simulink model "Zad1_Adasiak"  (R2020b)
settings: Solver=VariableStepAuto  StartTime=0.0  StopTime=0.0  RelTol=1e-3
undefined symbols (not defined in the file): H, W
libraries: CPOiS_SourcesSinks x10, CPOiS_LinearTransforms x4, CPOiS_DataManipulation_DataTypeConversion x4, CPOiS_General x1
settings Model: Creator=Krystian  LastModifiedBy=wadasiak

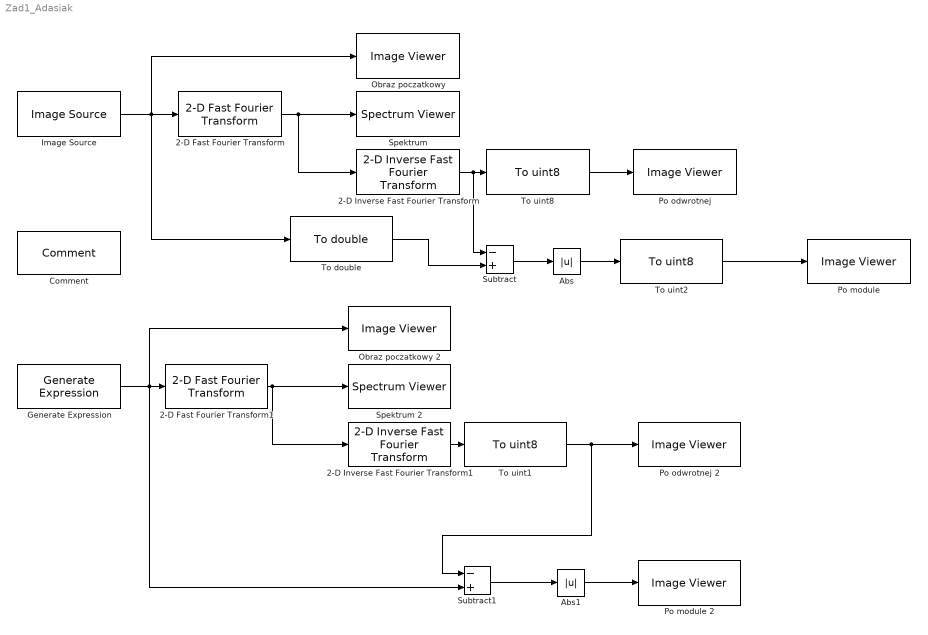
== system Zad1_Adasiak ==
  2-D Fast Fourier Transform : CPOiS_LinearTransforms/2-D Fast Fourier Transform
      settings: SourceProductName=CPOiS - Digital image and signal processing
  2-D Fast Fourier Transform1 : CPOiS_LinearTransforms/2-D Fast Fourier Transform
      settings: SourceProductName=CPOiS - Digital image and signal processing
  2-D Inverse Fast Fourier Transform : CPOiS_LinearTransforms/2-D Inverse Fast  Fourier Transform
      settings: SourceProductName=CPOiS - Digital image and signal processing
  2-D Inverse Fast Fourier Transform1 : CPOiS_LinearTransforms/2-D Inverse Fast  Fourier Transform
      settings: SourceProductName=CPOiS - Digital image and signal processing
  Abs : Abs
  Abs1 : Abs
  Comment : CPOiS_General/Comment
      settings: SourceProductName=CPOiS - Digital image and signal processing
  Generate Expression : CPOiS_SourcesSinks/Generate Expression  Width=256  Height=256  Expression=50.*(sin(W)+sin(2*H)+2)
      settings: SourceProductName=CPOiS - Digital image and signal processing
  Image Source : CPOiS_SourcesSinks/Image Source  FileSelection=marine.png
      settings: SourceProductName=CPOiS - Digital image and signal processing
  Obraz poczatkowy : CPOiS_SourcesSinks/Image Viewer
      settings: SourceProductName=CPOiS - Digital image and signal processing
  Obraz poczatkowy 2 : CPOiS_SourcesSinks/Image Viewer
      settings: SourceProductName=CPOiS - Digital image and signal processing
  Po module : CPOiS_SourcesSinks/Image Viewer
      settings: SourceProductName=CPOiS - Digital image and signal processing
  Po module 2 : CPOiS_SourcesSinks/Image Viewer
      settings: SourceProductName=CPOiS - Digital image and signal processing
  Po odwrotnej : CPOiS_SourcesSinks/Image Viewer
      settings: SourceProductName=CPOiS - Digital image and signal processing
  Po odwrotnej 2 : CPOiS_SourcesSinks/Image Viewer
      settings: SourceProductName=CPOiS - Digital image and signal processing
  Spektrum : CPOiS_SourcesSinks/Spectrum Viewer
      settings: SourceProductName=CPOiS - Digital image and signal processing
  Spektrum 2 : CPOiS_SourcesSinks/Spectrum Viewer
      settings: SourceProductName=CPOiS - Digital image and signal processing
  Subtract : Sum  Inputs=-+
  Subtract1 : Sum  Inputs=-+
  To double : CPOiS_DataManipulation_DataTypeConversion/To double
      settings: SourceProductName=CPOiS - Digital image and signal processing
  To uint1 : CPOiS_DataManipulation_DataTypeConversion/To uint8
      settings: SourceProductName=CPOiS - Digital image and signal processing
  To uint2 : CPOiS_DataManipulation_DataTypeConversion/To uint8
      settings: SourceProductName=CPOiS - Digital image and signal processing
  To uint8 : CPOiS_DataManipulation_DataTypeConversion/To uint8
      settings: SourceProductName=CPOiS - Digital image and signal processing
  wires:
  To uint1/1 -> Po odwrotnej 2/1, Subtract1/1
  Subtract1/1 -> Abs1/1
  Abs1/1 -> Po module 2/1
  Subtract/1 -> Abs/1
  Image Source/1 -> To double/1, Obraz poczatkowy/1, 2-D Fast Fourier Transform/1
  To uint8/1 -> Po odwrotnej/1
  2-D Inverse Fast Fourier Transform1/1 -> To uint1/1
  2-D Fast Fourier Transform1/1 -> Spektrum 2/1, 2-D Inverse Fast Fourier Transform1/1
  2-D Inverse Fast Fourier Transform/1 -> Subtract/1, To uint8/1
  Generate Expression/1 -> Subtract1/2, Obraz poczatkowy 2/1, 2-D Fast Fourier Transform1/1
  2-D Fast Fourier Transform/1 -> Spektrum/1, 2-D Inverse Fast Fourier Transform/1
  To double/1 -> Subtract/2
  Abs/1 -> To uint2/1
  To uint2/1 -> Po module/1
